simulink model "CHM2Ctrl"  (R2018b)
settings: Solver=FixedStepDiscrete  StartTime=0.0  StopTime=10.0  FixedStep=0.01  RelTol=1e-3
undefined symbols (not defined in the file or in its folder): KeSMSbMdChime2Enable_Val, KeSMSuChmReqDurnTm_Val, KeSMSuChmReqIntlTm_Val
libraries: RspLib x3
settings Model: Creator=sn2xws  LastModifiedBy=sn2xws
settings DataIOCC: SaveFormat=StructureWithTime
settings OptimizationCC: DefaultParameterBehavior=Inlined  EnhancedBackFolding=on  PassReuseOutputArgsAs=Individual arguments  ZeroExternalMemoryAtStartup=off  ZeroInternalMemoryAtStartup=off  OptimizeBlockOrder=speed  DifferentSizesBufferReuse=on  OptimizationCustomize=off
settings DebuggingCC: ParameterTunabilityLossMsg=error
settings ModelReferenceCC: ModelReferenceNumInstancesAllowed=Single
settings SFSimCC: MATLABDynamicMemAlloc=off
settings RTWCC: SystemTargetFile=autosar.tlc  GenCodeOnly=on  TemplateMakefile=ert_default_tmf  Description=AUTOSAR  GenerateReport=on  IncludeHyperlinkInReport=on  LaunchReport=on  GenerateTraceInfo=on  GenerateTraceReport=on  GenerateTraceReportSl=on  GenerateTraceReportSf=on  GenerateTraceReportEml=on
settings CodeAppCC: ForceParamTrailComments=on  IgnoreCustomStorageClasses=off  OperatorAnnotations=on  SimulinkDataObjDesc=on  SFDataObjDesc=on  InsertBlockDesc=on
settings STFCustomTargetCC: TargetLangStandard=C99 (ISO)  MultiwordLength=256  ParMdlRefBuildCompliant=on  CompOptLevelCompliant=on  IncludeMdlTerminateFcn=off  CombineOutputUpdateFcns=on  SuppressErrorStatus=on  ERTCustomFileBanners=on  SupportNonFinite=off  SupportComplex=off  SupportContinuousTime=off  SupportNonInlinedSFcns=off  RemoveResetFunc=on  MATLABClassNameForMDSCustomization=Simulink.SoftwareTarget.ERTCustomization  AutosarCompliant=on  UseToolchainInfoCompliant=on  LookupTableObjectStructAxisOrder=2,1,3,4,...  LUTObjectStructOrderEvenSpacing=Size,Table,Breakpoints  SystemTargetFile=autosar.tlc
settings ERTTargetCC: TargetLangStandard=C99 (ISO)  ConcurrentExecutionCompliant=off  IncludeMdlTerminateFcn=off  SuppressErrorStatus=on  SupportNonFinite=off  SupportComplex=off  ModelStepFunctionPrototypeControlCompliant=off  CPPClassGenCompliant=off  AutosarCompliant=on  LookupTableObjectStructAxisOrder=2,1,3,4,...  LUTObjectStructOrderEvenSpacing=Size,Table,Breakpoints  InlinedParameterPlacement=NonHierarchical  ERTCustomFileTemplate=example_file_process.tlc

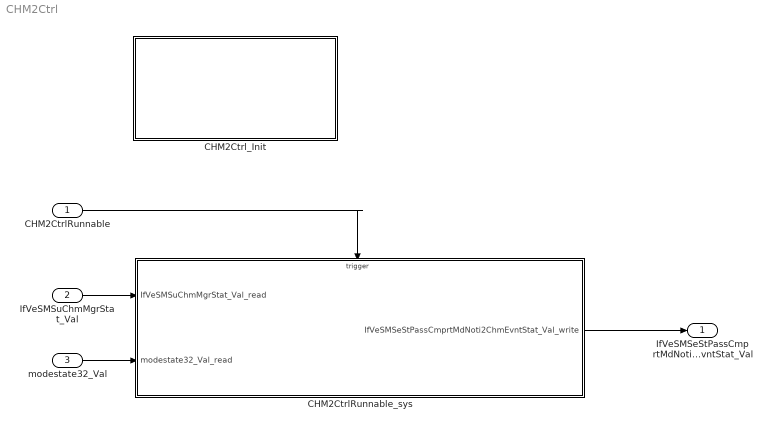
== system CHM2Ctrl ==
  CHM2CtrlRunnable : Inport  SampleTime=0.01  OutputFunctionCall=on
  IfVeSMSuChmMgrStat_Val : Inport  Port=2  OutDataTypeStr=uint16  PortDimensions=1
  modestate32_Val : Inport  Port=3  OutDataTypeStr=uint32  PortDimensions=1
  CHM2CtrlRunnable_sys : Subsystem
  CHM2Ctrl_Init : Subsystem
  IfVeSMSeStPassCmprtMdNoti2ChmEvntStat_Val : Outport  OutDataTypeStr=Enum: EventSts1  PortDimensions=1
  wires:
  IfVeSMSuChmMgrStat_Val/1 -> CHM2CtrlRunnable_sys/1(IfVeSMSuChmMgrStat_Val_read)
  modestate32_Val/1 -> CHM2CtrlRunnable_sys/2(modestate32_Val_read)
  CHM2CtrlRunnable_sys/1(IfVeSMSeStPassCmprtMdNoti2ChmEvntStat_Val_write) -> IfVeSMSeStPassCmprtMdNoti2ChmEvntStat_Val/1
  CHM2CtrlRunnable/1 -> CHM2CtrlRunnable_sys/Trigger

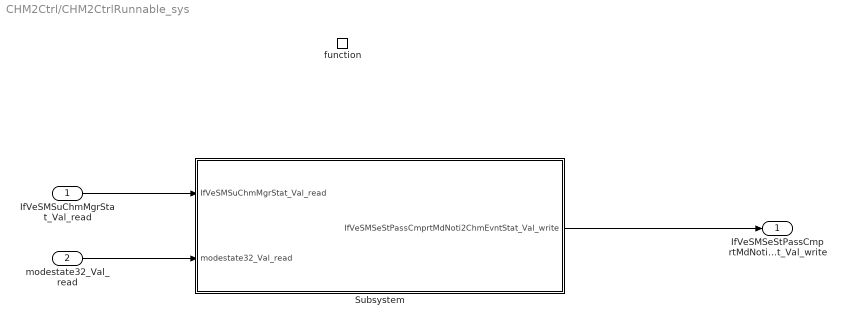
== system CHM2Ctrl/CHM2CtrlRunnable_sys ==
  IfVeSMSuChmMgrStat_Val_read : Inport
  modestate32_Val_read : Inport  Port=2
  function : TriggerPort  TriggerType=function-call  VariantControl=(inherit)  SampleTimeType=periodic  SampleTime=-1
  Subsystem : Subsystem
  IfVeSMSeStPassCmprtMdNoti2ChmEvntStat_Val_write : Outport
      settings: EnsureOutportIsVirtual=on
  wires:
  IfVeSMSuChmMgrStat_Val_read/1 -> Subsystem/1(IfVeSMSuChmMgrStat_Val_read)
  modestate32_Val_read/1 -> Subsystem/2(modestate32_Val_read)
  Subsystem/1(IfVeSMSeStPassCmprtMdNoti2ChmEvntStat_Val_write) -> IfVeSMSeStPassCmprtMdNoti2ChmEvntStat_Val_write/1

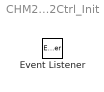
== system CHM2Ctrl/CHM2Ctrl_Init ==
  Event Listener : EventListener  EventName=reset

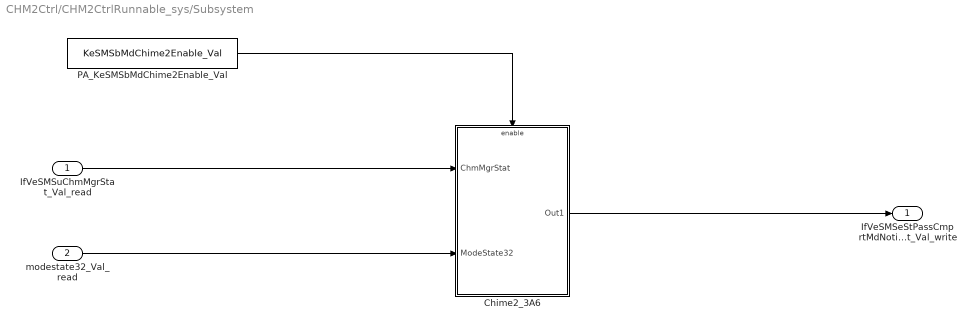
== system CHM2Ctrl/CHM2CtrlRunnable_sys/Subsystem ==
  IfVeSMSuChmMgrStat_Val_read : Inport
  modestate32_Val_read : Inport  Port=2
  Chime2_3A6 : Subsystem
  PA_KeSMSbMdChime2Enable_Val : Constant  Value=KeSMSbMdChime2Enable_Val
  IfVeSMSeStPassCmprtMdNoti2ChmEvntStat_Val_write : Outport
      settings: EnsureOutportIsVirtual=on
  wires:
  modestate32_Val_read/1 -> Chime2_3A6/2(ModeState32)
  PA_KeSMSbMdChime2Enable_Val/1 -> Chime2_3A6/Enable
  IfVeSMSuChmMgrStat_Val_read/1 -> Chime2_3A6/1(ChmMgrStat)
  Chime2_3A6/1(Out1) -> IfVeSMSeStPassCmprtMdNoti2ChmEvntStat_Val_write/1

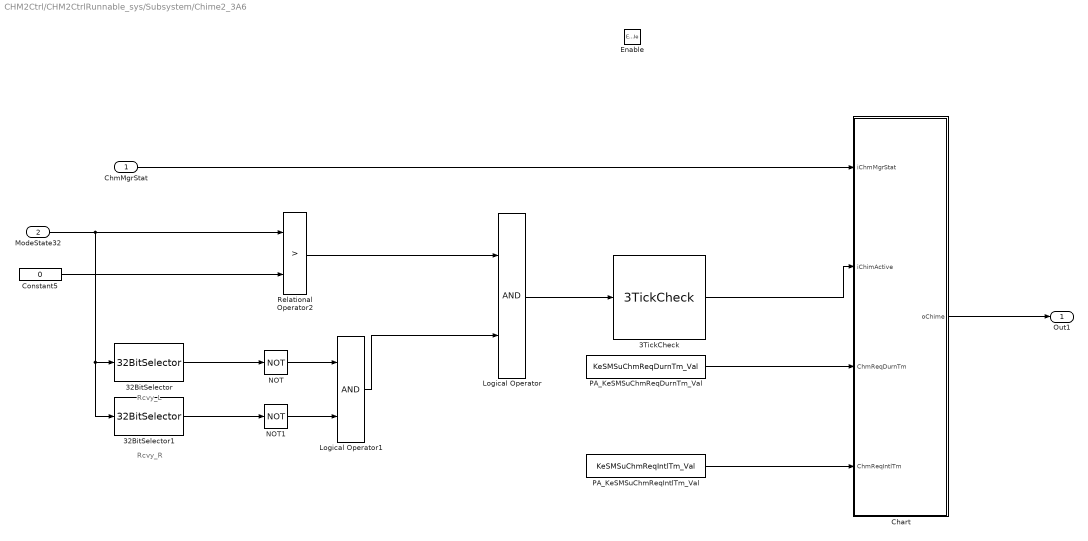
== system CHM2Ctrl/CHM2CtrlRunnable_sys/Subsystem/Chime2_3A6 ==
  note: Rcvy_L
  note: Rcvy_R
  ChmMgrStat : Inport
  ModeState32 : Inport  Port=2
  Enable : EnablePort
  32BitSelector : RspLib/32BitSelector  BitNum=10
  32BitSelector1 : RspLib/32BitSelector  BitNum=12
  3TickCheck : RspLib/3TickCheck  SystemSampleTime=-1
  Chart : Stateflow chart  TreatAsAtomicUnit=on
  Constant5 : Constant  Value=0  OutDataTypeStr=uint32
  Logical Operator : Logic  AllPortsSameDT=off  OutDataTypeStr=boolean
  Logical Operator1 : Logic  AllPortsSameDT=off  OutDataTypeStr=boolean
  NOT : Logic  Operator=NOT  AllPortsSameDT=off  OutDataTypeStr=boolean
  NOT1 : Logic  Operator=NOT  AllPortsSameDT=off  OutDataTypeStr=boolean
  PA_KeSMSuChmReqDurnTm_Val : Constant  Value=KeSMSuChmReqDurnTm_Val
  PA_KeSMSuChmReqIntlTm_Val : Constant  Value=KeSMSuChmReqIntlTm_Val
  Relational Operator2 : RelationalOperator  Operator=>  OutDataTypeStr=boolean  RndMeth=Simplest
  Out1 : Outport
  wires:
  ChmMgrStat/1 -> Chart/1(iChmMgrStat)
  Chart/1(oChime) -> Out1/1
  3TickCheck/1 -> Chart/2(iChimActive)
  Constant5/1 -> Relational Operator2/2
  ModeState32/1 -> 32BitSelector1/1, 32BitSelector/1, Relational Operator2/1
  Relational Operator2/1 -> Logical Operator/1
  Logical Operator/1 -> 3TickCheck/1
  Logical Operator1/1 -> Logical Operator/2
  NOT/1 -> Logical Operator1/1
  NOT1/1 -> Logical Operator1/2
  PA_KeSMSuChmReqDurnTm_Val/1 -> Chart/3(ChmReqDurnTm)
  PA_KeSMSuChmReqIntlTm_Val/1 -> Chart/4(ChmReqIntlTm)
  32BitSelector/1 -> NOT/1
  32BitSelector1/1 -> NOT1/1

== stateflow chart CHM2Ctrl/CHM2CtrlRunnable_sys/Subsystem/Chime2_3A6/Chart ==
  state CheckStat
    en:retrycnt=0;
    state Idle
      en:
      oChime = EventSts1.EventSts_NoAct;
    state Active1
      en:
      oChime = EventSts1.EventSts_Act;
    (default) -> CheckStat.Idle
    Active1 -> CheckStat.Idle [order 2] : [iChmMgrStat==2725||...
        | iChmMgrStat==0]
    Active1 -> CheckStat.Idle [order 1] : [after(ChmReqDurnTm/10,tick)]
        | {retrycnt=retrycnt+1;}
    CheckStat.Idle -> Active1 : [iChmMgrStat !=0&&iChmMgrStat!=2725&&retrycnt<4&&after(ChmReqIntlTm/10,tick)]
  state Idle
    en:
    oChime = EventSts1.EventSts_NoAct;
  state Cancel
    en:oChime = EventSts1.EventSts_CancleChime;
  state CancelwithNoCancel
    en:oChime = EventSts1.EventSts_NoAct;
  note: $0=NO_ACTION; $1=ACTIVE; $2=CANCEL_CHIME
  CheckStat -> CheckStat [order 3] : [hasChanged(iChmMgrStat)&&iChmMgrStat!=0&&iChmMgrStat!=2725]
  (default) -> Idle
  Idle -> CheckStat : [iChimActive]
  Cancel -> Idle : [after(ChmReqDurnTm/10,tick)]
  CheckStat -> Cancel [order 1] : [!iChimActive&&iChmMgrStat==2725]
  CancelwithNoCancel -> Cancel [order 2] : [iChmMgrStat==2725]
  CancelwithNoCancel -> Idle [order 1] : [after(ChmReqDurnTm/10,tick)]
  CheckStat -> CancelwithNoCancel [order 2] : [!iChimActive]
  data: iChmMgrStat input; iChimActive input boolean; oChime output Enum: EventSts1; retrycnt local uint8; ChmReqDurnTm input uint8; ChmReqIntlTm input uint8
